simulink model "fillingSystem"  (R2020b)
settings: Solver=VariableStepAuto  StartTime=0.0  StopTime=120  RelTol=1e-3  AbsTol=1e-3
undefined symbols (not defined in the file or in its folder): Sim
libraries: fl_lib x18, nesl_utility x8, pid_lib x1, SimscapeFluids_lib x1, simulink x1
settings Model: PacingRate=4  Creator=luc  LastModifiedBy=luc
settings SolverCC: AutoScaleAbsTol=off
settings DebuggingCC: SymbolicDimsDataTypeCodeGenerationDiagnostic=none
settings SFSimCC: CustomCodeUndefinedFunction=UseInterfaceOnly
settings SimscapeCC: SimscapeLogType=all  SimscapeLogSimulationStatistics=on  SimscapeLogDataHistory=10000

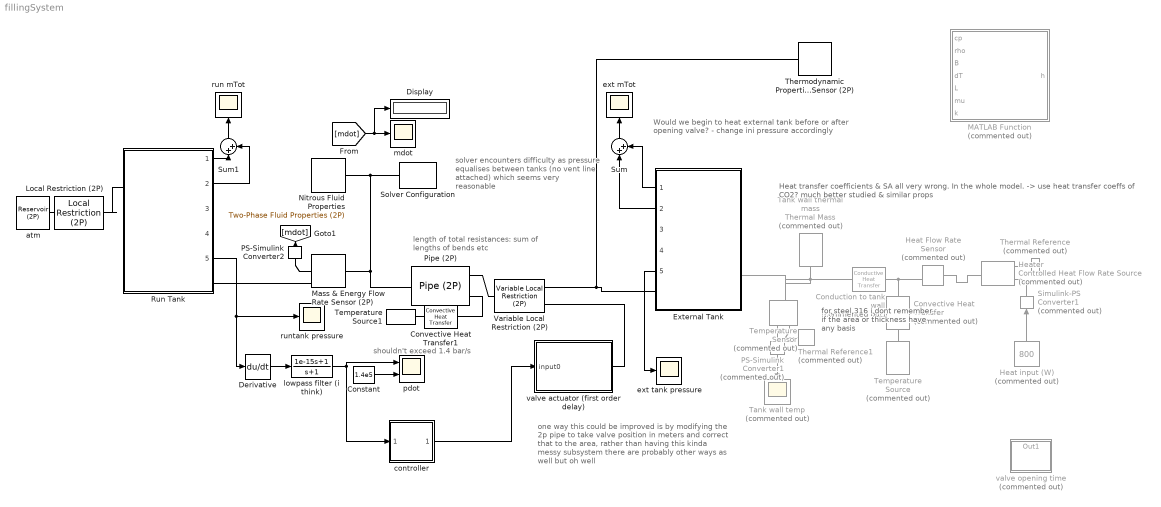
== system fillingSystem ==
  note: one way this could be improved is by modifying
      | the 2p pipe to take valve position in meters and
      | correct that to the area, rather than having this kinda messy subsystem
      |
      | there are probably other ways as well but oh well
  note: for steel 316
      | i dont remember if the area or thickness have any basis
  note: shouldn't exceed 1.4 bar/s
  note: solver encounters difficulty as
      |  pressure equalises between tanks
      | (no vent line attached) which seems
      | very reasonable
  note: Would we begin to heat external tank before or after
      | opening valve? - change ini pressure accordingly
  note: length of total resistances: sum of lengths of bends etc
  note: Heat transfer coefficients & SA all very wrong. In the whole model.
      | -> use heat transfer coeffs of CO2? much better studied & similar props
  Conduction to tank wall : fl_lib/Thermal/Thermal Elements/Conductive Heat Transfer  Commented=on  area=0.63 m^2  thickness=2.2e-3 m  th_cond=16 W/(m*K)  T_specify=off  T_priority=None  T=0 K  T_nominal_specify=off  T_nominal_unit=K  T_nominal_value=1  Q_specify=off  Q_priority=None  Q=0 W  Q_nominal_specify=off  Q_nominal_unit=W  Q_nominal_value=1
  Constant : Constant  Value=1.4e5
  Convective Heat Transfer : fl_lib/Thermal/Thermal Elements/Convective Heat Transfer  Commented=on  area=0.1 m^2  heat_tr_coeff=20 W/(m^2 * K)  T_specify=off  T_priority=None  T=0 K  T_nominal_specify=off  T_nominal_unit=K  T_nominal_value=1  Q_specify=off  Q_priority=None  Q=0 W  Q_nominal_specify=off  Q_nominal_unit=W  Q_nominal_value=1
  Convective Heat Transfer1 : fl_lib/Thermal/Thermal Elements/Convective Heat Transfer  area=3e-4 m^2  heat_tr_coeff=20 W/(m^2 * K)  T_specify=off  T_priority=None  T=0 K  T_nominal_specify=off  T_nominal_unit=K  T_nominal_value=1  Q_specify=off  Q_priority=None  Q=0 W  Q_nominal_specify=off  Q_nominal_unit=W  Q_nominal_value=1
  Derivative : Derivative
  Display : Display
  External Tank : Subsystem  ReferencedSubsystem=Nitrous_Tank_Custom  nitrousLiqConCrossSection=Sim.fillpipe.crossSection  nitrousVapConCrossSection=2e-5  nitrousTankVol=Sim.extTank.volume  initialTankPressure=Sim.extTank.pressure  initialLiqMassFraction=0.7  totalHeatTransferSurfaceArea=6  heatTranferWallToLiq=100  heatTranferWallToVap=15.5
  Heat Flow Rate Sensor : fl_lib/Thermal/Thermal Sensors/Heat Flow Rate Sensor  Commented=on
      settings: SourceProductBaseCode=SS
  Heat input (W) : Constant  Commented=on  Value=800
  Heater : fl_lib/Thermal/Thermal Sources/Controlled Heat Flow Rate Source  Commented=on
  Local Restriction (2P) : fl_lib/Two-Phase Fluid/Elements/Local Restriction (2P)  restriction_area=1e-6 m^2  area=0.01 m^2  Cd=0.64  B_lam=0.999
      settings: SourceProductBaseCode=SS  InternalSimscapePortConfiguration="{\"Bottom\":[],\"Left\":[{\"id\":\"A\",\"label\":\"A\",\"type\":\"foundation.two_phase_fluid.two_phase_fluid\"}],\"Right\":[{\"id\":\"B\",\"label\":\"B\",\"type\":\"foundation.two_phase_fluid.two_phase_fluid\"}],\"Top\":[]}"
  MATLAB Function : MATLAB Function  Commented=on  TreatAsAtomicUnit=on
  Mass & Energy Flow Rate Sensor (2P) : fl_lib/Two-Phase Fluid/Sensors/Mass & Energy Flow Rate Sensor (2P)
      settings: SourceProductBaseCode=SS  InternalSimscapePortConfiguration="{\"Bottom\":[],\"Left\":[{\"id\":\"A\",\"label\":\"A\",\"type\":\"foundation.two_phase_fluid.two_phase_fluid\"}],\"Right\":[{\"id\":\"B\",\"label\":\"B\",\"type\":\"foundation.two_phase_fluid.two_phase_fluid\"},{\"id\":\"M\",\"label\":\"M\",\"type\":\"output\"},{\"id\":\"PHI\",\"label\":\"Phi\",\"type\":\"output\"}],\"Top\":[]}"
  Nitrous Fluid Properties : fl_lib/Two-Phase Fluid/Utilities/Two-Phase Fluid Properties (2P)  u_min=Sim.nitrousFluidTable.u_min kJ/kg  u_max=Sim.nitrousFluidTable.u_max kJ/kg  unorm_liq=Sim.nitrousFluidTable.liquid.unorm  unorm_vap=Sim.nitrousFluidTable.vapor.unorm  p_TLU=Sim.nitrousFluidTable.p MPa  v_liq=Sim.nitrousFluidTable.liquid.v m^3/kg  v_vap=Sim.nitrousFluidTable.vapor.v m^3/kg  s_liq=Sim.nitrousFluidTable.liquid.s kJ/kg/K  s_vap=Sim.nitrousFluidTable.vapor.s kJ/kg/K  T_liq=Sim.nitrousFluidTable.liquid.T K  T_vap=Sim.nitrousFluidTable.vapor.T K  nu_liq=Sim.nitrousFluidTable.liquid.nu mm^2/s  nu_vap=Sim.nitrousFluidTable.vapor.nu mm^2/s  k_liq=Sim.nitrousFluidTable.liquid.k W/(m*K)  k_vap=Sim.nitrousFluidTable.vapor.k W/(m*K)  Pr_liq=Sim.nitrousFluidTable.liquid.Pr  Pr_vap=Sim.nitrousFluidTable.vapor.Pr  u_sat_liq=Sim.nitrousFluidTable.liquid.u_sat kJ/kg  u_sat_vap=Sim.nitrousFluidTable.vapor.u_sat kJ/kg  p_crit=Sim.nitrousFluidTable.p_crit MPa  critical_region=foundation.enum.critical_region.clip  p_crit_fraction=0.12  p_atm=0.101325 MPa  q_rev=0.01 Pa
      settings: SourceProductBaseCode=SS  InternalSimscapePortConfiguration="{\"Bottom\":[],\"Left\":[],\"Right\":[{\"id\":\"A\",\"label\":\"\",\"type\":\"foundation.two_phase_fluid.two_phase_fluid\"}],\"Top\":[]}"
  PS-Simulink Converter1 : nesl_utility/PS-Simulink Converter  Commented=on  PhysicalDomain=network_engine_domain  SubClassName=ps_output  LeftPortType=input  RightPortType=output  PseudoPeriodic=off  Frequencies=[]  Unit=inherit  AffineConversion=off
  PS-Simulink Converter2 : nesl_utility/PS-Simulink Converter  PhysicalDomain=network_engine_domain  SubClassName=ps_output  LeftPortType=input  RightPortType=output  PseudoPeriodic=off  Frequencies=[]  Unit=inherit  AffineConversion=off
  Pipe (2P) : fl_lib/Two-Phase Fluid/Elements/Pipe (2P)  length=1 m  area=Sim.fillpipe.crossSection m^2  Dh=Sim.fillpipe.diameter m  length_add=1 m  roughness=Sim.fillpipe.roughness m  Re_lam=2000  Re_tur=4000  shape_factor=64  Nu_lam=3.66  inertia=simscape.enum.onoff.off  energy_spec=foundation.enum.energy_spec.quality  p_init=1.05e5 Pa  T_init=25 degC  x_init=1  alpha_init=0.1  h_init=1500 kJ/kg  u_init=1500 kJ/kg  mdot_init=0 kg/s  time_constant=0.01 s
      settings: SourceProductBaseCode=SS  InternalSimscapePortConfiguration="{\"Bottom\":[],\"Left\":[{\"id\":\"A\",\"label\":\"A\",\"type\":\"foundation.two_phase_fluid.two_phase_fluid\"},{\"id\":\"H\",\"label\":\"H\",\"type\":\"foundation.thermal.thermal\"}],\"Right\":[{\"id\":\"B\",\"label\":\"B\",\"type\":\"foundation.two_phase_fluid.two_phase_fluid\"}],\"Top\":[]}"
  Run Tank : Subsystem  ReferencedSubsystem=Nitrous_Tank_Custom  nitrousLiqConCrossSection=Sim.fillpipe.crossSection  nitrousVapConCrossSection=2e-5  nitrousTankVol=Sim.runTank.volume  initialTankPressure=Sim.PAmbient  initialLiqMassFraction=0.01  totalHeatTransferSurfaceArea=6  heatTranferWallToLiq=10  heatTranferWallToVap=10
  Simulink-PS Converter1 : nesl_utility/Simulink-PS Converter  Commented=on  PhysicalDomain=network_engine_domain  SubClassName=ps_input  LeftPortType=input  RightPortType=output  PseudoPeriodic=off  Frequencies=[]  NoiseDistribution=none  NoiseParameters=[]  Unit=1  AffineConversion=off  FilteringAndDerivatives=provide  SimscapeFilterOrder=1  InputFilterTimeConstant=0.001  UdotUserProvided=0
  Solver Configuration : nesl_utility/Solver Configuration  PhysicalDomain=network_engine_domain  SubClassName=solver  LeftPortType=input  RightPortType=generic  Tones=[]  Harmonics=[]  SimulateNoise=off  Profile=off  UseLocalSampling=off  EnableSwitchedLinearOptims=on  FrequencyDomain=off  UseCCode=off  RelTol=0.001  AbsTol=1e-06  MinStep=1e-09  ToWorkspace=off  RevertToSquareIcSolve=off  NumHomotopyIterations=100  PhasorMode=off  PhasorModeNumHarmonics=1  DoDC=off  ResidualTolerance=1e-09  UseLocalSolver=off  LocalSolverChoice=NE_BACKWARD_EULER_ADVANCER  LocalSolverSampleTime=0.001  DoFixedCost=off  MaxNonlinIter=3  MaxModeIter=2  ComputeImpulses=off  ImpulseIterations=2  LinearAlgebra=auto  EquationFormulation=NE_TIME_EF  DelaysMemoryBudget=1024  AutomaticFiltering=on  FilteringTimeConstant=0.001  PartitionStorageMethod=AS_NEEDED  PartitionMemoryBudget=1024  PartitionMethod=ROBUST
      settings: SourceProductName=Utilities
  Sum : Sum  Inputs=|++
  Sum1 : Sum  Inputs=|++
  Tank wall thermal mass : fl_lib/Thermal/Thermal Elements/Thermal Mass  Commented=on  mass=6 kg  sp_heat=500 J/kg/K  T_specify=on  T_priority=High  T=300 K  T_nominal_specify=off  T_nominal_unit=K  T_nominal_value=1  Q_specify=off  Q_priority=None  Q=0 W  Q_nominal_specify=off  Q_nominal_unit=W  Q_nominal_value=1
  Tank wall temp : Scope  Commented=on
  Temperature Sensor : fl_lib/Thermal/Thermal Sensors/Temperature Sensor  Commented=on
  Temperature Source : fl_lib/Thermal/Thermal Sources/Temperature Source  Commented=on  temperature=293.15 K
  Temperature Source1 : fl_lib/Thermal/Thermal Sources/Temperature Source  temperature=293.15 K
  Thermal Reference : fl_lib/Thermal/Thermal Elements/Thermal Reference  Commented=on
  Thermal Reference1 : fl_lib/Thermal/Thermal Elements/Thermal Reference  Commented=on
  Thermodynamic Properties Sensor (2P) : fl_lib/Two-Phase Fluid/Sensors/Thermodynamic Properties Sensor (2P)
      settings: SourceProductBaseCode=SS  InternalSimscapePortConfiguration="{\"Bottom\":[],\"Left\":[{\"id\":\"A\",\"label\":\"A\",\"type\":\"foundation.two_phase_fluid.two_phase_fluid\"}],\"Right\":[{\"id\":\"T\",\"label\":\"T\",\"type\":\"output\"},{\"id\":\"H\",\"label\":\"h\",\"type\":\"output\"},{\"id\":\"V\",\"label\":\"v\",\"type\":\"output\"},{\"id\":\"S\",\"label\":\"s\",\"type\":\"output\"}],\"Top\":[]}"
  Variable Local Restriction (2P) : fl_lib/Two-Phase Fluid/Elements/Variable Local Restriction (2P)  min_area=1e-12 m^2  max_area=Sim.controlValve.crossSection m^2  area=Sim.fillpipe.diameter m^2  Cd=0.64  B_lam=0.999
      settings: SourceProductBaseCode=SS  InternalSimscapePortConfiguration="{\"Bottom\":[],\"Left\":[{\"id\":\"A\",\"label\":\"A\",\"type\":\"foundation.two_phase_fluid.two_phase_fluid\"},{\"id\":\"area_in\",\"label\":\"AR\",\"type\":\"input\"}],\"Right\":[{\"id\":\"B\",\"label\":\"B\",\"type\":\"foundation.two_phase_fluid.two_phase_fluid\"}],\"Top\":[]}"
  atm : fl_lib/Two-Phase Fluid/Elements/Reservoir (2P)  pressure_spec=foundation.enum.pressure_spec.atmospheric  reservoir_pressure=0.101325 MPa  energy_spec=foundation.enum.energy_spec.temperature  reservoir_temperature=293.15 K  reservoir_quality=0.5  reservoir_void_fraction=0.5  reservoir_enthalpy=1500 kJ/kg  reservoir_internal_energy=1500 kJ/kg  area_A=5e-7 m^2
      settings: SourceProductBaseCode=SS
  controller : Subsystem
  ext mTot : Scope
  ext tank pressure : Scope
  lowpass filter (i think) : TransferFcn  Numerator=[1e-15, 1]  Denominator=[1 1]
  mdot : Scope
  pdot : Scope  NumInputPorts=2
  run mTot : Scope
  runtank pressure : Scope
  valve actuator (first order delay) : Subsystem
  valve opening time : Subsystem  Commented=on
  wires:
  Heat input (W)/1 -> Simulink-PS Converter1/1
  Sum/1 -> ext mTot/1
  Sum1/1 -> run mTot/1
  PS-Simulink Converter1/1 -> Tank wall temp/1
  PS-Simulink Converter2/1 -> [mdot]
  [mdot] -> Display/1, mdot/1
  Run Tank/5 -> Derivative/1, runtank pressure/1
  External Tank/5 -> ext tank pressure/1
  External Tank/1 -> Sum/2
  External Tank/2 -> Sum/1
  Run Tank/1 -> Sum1/1
  Run Tank/2 -> Sum1/2
  Derivative/1 -> lowpass filter (i think)/1
  lowpass filter (i think)/1 -> controller/1(pdot), pdot/1
  controller/1(Output) -> valve actuator (first order delay)/1(input0)
  Constant/1 -> pdot/2
  connections:
  Variable Local Restriction (2P)/LConn1 -- Thermodynamic Properties Sensor (2P)/LConn1 -- External Tank/RConn1
  Conduction to tank wall/RConn1 -- Temperature Sensor/LConn1 -- External Tank/LConn2 -- Tank wall thermal mass/LConn1
  Convective Heat Transfer/LConn1 -- Heat Flow Rate Sensor/RConn2 -- Conduction to tank wall/LConn1
  Thermal Reference/LConn1 -- Heater/RConn2
  Simulink-PS Converter1/RConn1 -- Heater/RConn1
  Thermal Reference1/LConn1 -- Temperature Sensor/RConn1
  PS-Simulink Converter1/LConn1 -- Temperature Sensor/RConn2
  Convective Heat Transfer/RConn1 -- Temperature Source/LConn1
  Mass & Energy Flow Rate Sensor (2P)/RConn2 -- PS-Simulink Converter2/LConn1
  Convective Heat Transfer1/RConn1 -- Temperature Source1/LConn1
  Pipe (2P)/LConn2 -- Convective Heat Transfer1/LConn1
  Nitrous Fluid Properties/RConn1 -- Solver Configuration/RConn1 -- Pipe (2P)/RConn1 -- Mass & Energy Flow Rate Sensor (2P)/LConn1
  Heat Flow Rate Sensor/LConn1 -- Heater/LConn1
  Pipe (2P)/LConn1 -- Variable Local Restriction (2P)/RConn1
  Run Tank/RConn1 -- Mass & Energy Flow Rate Sensor (2P)/RConn1
  Local Restriction (2P)/LConn1 -- atm/LConn1
  Local Restriction (2P)/RConn1 -- Run Tank/LConn1
  valve actuator (first order delay)/RConn1 -- Variable Local Restriction (2P)/LConn2

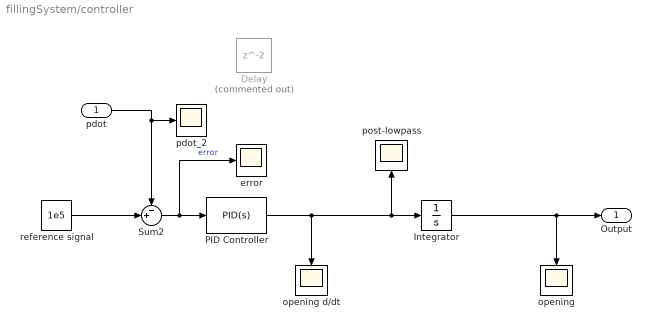
== system fillingSystem/controller ==
  pdot : Inport
  Delay : Delay  Commented=on
  Integrator : Integrator  InitialCondition=0.05  LimitOutput=on  UpperSaturationLimit=1  LowerSaturationLimit=0.05
  PID Controller : pid_lib/PID Controller  Controller=PID  Form=Parallel  TimeDomain=Continuous-time  UseExternalTs=off  SampleTime=-1  IntegratorMethod=Forward Euler  FilterMethod=Forward Euler  ControllerParametersSource=internal  P=2e-5  I=1e-5  D=6e-5  UseFilter=on  N=100  TunerSelectOption=Transfer Function Based (PID Tuner App)  InitialConditionSource=internal  InitialConditionForIntegrator=0  InitialConditionForFilter=0  DifferentiatorICPrevScaledInput=0  ExternalReset=none  TrackingMode=off  Kt=1  LimitOutput=off  SatLimitsSource=internal  UpperSaturationLimit=1  LowerSaturationLimit=0  LinearizeAsGain=on  AntiWindupMode=none  Kb=1  POutMin=[]  POutMax=[]  IOutMin=[]  IOutMax=[]  DOutMin=[]  DOutMax=[]  NOutMin=[]  NOutMax=[]  SumOutMin=[]  SumOutMax=[]  SaturationOutMin=[]  SaturationOutMax=[]  PParamMin=[]  PParamMax=[]  IParamMin=[]  IParamMax=[]  DParamMin=[]  DParamMax=[]  NParamMin=[]  NParamMax=[]  KbParamMin=[]  KbParamMax=[]  KtParamMin=[]  KtParamMax=[]  KbOutMin=[]  KbOutMax=[]  KtOutMin=[]  KtOutMax=[]  IntegratorOutMin=[]  IntegratorOutMax=[]  FilterOutMin=[]  FilterOutMax=[]  SumI1OutMin=[]  SumI1OutMax=[]  SumI2OutMin=[]  SumI2OutMax=[]  SumI3OutMin=[]  SumI3OutMax=[]  SumI4OutMin=[]  SumI4OutMax=[]  SumDOutMin=[]  SumDOutMax=[]  DifferentiatorOutMin=[]  DifferentiatorOutMax=[]  FilterDiffOutCoefMin=[]  FilterDiffOutCoefMax=[]  ReciprocalOutMin=[]  ReciprocalOutMax=[]  SumDenOutMin=[]  SumDenOutMax=[]  SumNumOutMin=[]  SumNumOutMax=[]  DivideOutMin=[]  DivideOutMax=[]  UdiffTsProdOutMin=[]  UdiffTsProdOutMax=[]  NTsProdOutMin=[]  NTsProdOutMax=[]  UintegralTsProdOutMin=[]  UintegralTsProdOutMax=[]  UngainTsProdOutMin=[]  UngainTsProdOutMax=[]  IntegratorContinuousStateAttributes=''  IntegratorStateMustResolveToSignalObject=off  IntegratorRTWStateStorageClass=Auto  FilterContinuousStateAttributes=''  FilterStateMustResolveToSignalObject=off  FilterRTWStateStorageClass=Auto  ParallelPVariant=InternalParameters  IdealPVariant=Disabled  IVariant=InternalParameters  DVariant=InternalParameters  IntegratorVariant=Continuous  SatVariant=Disabled  AWVariant=Passthrough  PCopyVariant=Disabled  TRVariant=Disabled  FdbkBlocksVariant=Forward  IdealPFdbkVariant=Disabled  SatFdbkVariant=Disabled  DerivativeFilterVariant=ContFilter  NVariant=InternalParameters  NCopyVariant=Disabled  FilterICVariant=InternalICsFilter  IntegratorICVariant=InternalICs  ExternalResetVariant=Disabled  TRSumVariant=Passthrough  SumFdbkVariant=Disabled  SumVariant=Sum_PID  TsampFilterVariant=InternalTs  TsampNgainVariant=Passthrough  TsampIntegralVariant=Passthrough  ExternalSaturationOutDataTypeStr=Inherit: Same as second input
  Sum2 : Sum  Inputs=-+|
  error : Scope
  opening : Scope
  opening d/dt : Scope
  pdot_2 : Scope
  post-lowpass : Scope
  reference signal : Constant  Value=1e5
  Output : Outport
  wires:
  reference signal/1 -> Sum2/2
  pdot/1 -> Sum2/1, pdot_2/1
  Sum2/1 -> error/1, PID Controller/1  "error"
  PID Controller/1 -> post-lowpass/1, Integrator/1, opening d/dt/1
  Integrator/1 -> Output/1, opening/1

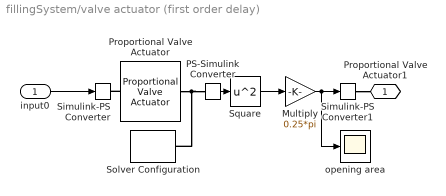
== system fillingSystem/valve actuator (first order delay) ==
  input0 : Inport
  Multiply : Gain  Gain=0.25*pi
  PS-Simulink Converter : nesl_utility/PS-Simulink Converter  PhysicalDomain=network_engine_domain  SubClassName=ps_output  LeftPortType=input  RightPortType=output  PseudoPeriodic=off  Frequencies=[]  Unit=inherit  AffineConversion=off
  Proportional Valve Actuator : SimscapeFluids_lib/Valve Actuators/Proportional Valve Actuator  gain=Sim.controlValve.diameter m  time_constant=8 s  valve_stroke=Sim.controlValve.diameter m
      settings: SourceProductBaseCode=SH  InternalSimscapePortConfiguration="{\"Bottom\":[],\"Left\":[{\"id\":\"A\",\"label\":\"A\",\"type\":\"input\"}],\"Right\":[{\"id\":\"S\",\"label\":\"S\",\"type\":\"output\"}],\"Top\":[]}"
  Simulink-PS Converter : nesl_utility/Simulink-PS Converter  PhysicalDomain=network_engine_domain  SubClassName=ps_input  LeftPortType=input  RightPortType=output  PseudoPeriodic=off  Frequencies=[]  NoiseDistribution=none  NoiseParameters=[]  Unit=1  AffineConversion=off  FilteringAndDerivatives=provide  SimscapeFilterOrder=1  InputFilterTimeConstant=0.001  UdotUserProvided=0
  Simulink-PS Converter1 : nesl_utility/Simulink-PS Converter  PhysicalDomain=network_engine_domain  SubClassName=ps_input  LeftPortType=input  RightPortType=output  PseudoPeriodic=off  Frequencies=[]  NoiseDistribution=none  NoiseParameters=[]  Unit=1  AffineConversion=off  FilteringAndDerivatives=provide  SimscapeFilterOrder=1  InputFilterTimeConstant=0.001  UdotUserProvided=0
  Solver Configuration : nesl_utility/Solver Configuration  PhysicalDomain=network_engine_domain  SubClassName=solver  LeftPortType=input  RightPortType=generic  Tones=[]  Harmonics=[]  SimulateNoise=off  Profile=off  UseLocalSampling=off  EnableSwitchedLinearOptims=on  FrequencyDomain=off  UseCCode=off  RelTol=0.001  AbsTol=1e-06  MinStep=1e-09  ToWorkspace=off  RevertToSquareIcSolve=off  NumHomotopyIterations=100  PhasorMode=off  PhasorModeNumHarmonics=1  DoDC=off  ResidualTolerance=1e-09  UseLocalSolver=off  LocalSolverChoice=NE_BACKWARD_EULER_ADVANCER  LocalSolverSampleTime=0.001  DoFixedCost=off  MaxNonlinIter=3  MaxModeIter=2  ComputeImpulses=off  ImpulseIterations=2  LinearAlgebra=auto  EquationFormulation=NE_TIME_EF  DelaysMemoryBudget=1024  AutomaticFiltering=on  FilteringTimeConstant=0.001  PartitionStorageMethod=AS_NEEDED  PartitionMemoryBudget=1024  PartitionMethod=ROBUST
  Square : Math  Operator=square  SaturateOnIntegerOverflow=on
  opening area : Scope
  Proportional Valve Actuator1 : PMIOPort  Side=Right
  wires:
  input0/1 -> Simulink-PS Converter/1
  Multiply/1 -> opening area/1, Simulink-PS Converter1/1
  Square/1 -> Multiply/1
  PS-Simulink Converter/1 -> Square/1
  connections:
  Proportional Valve Actuator/LConn1 -- Simulink-PS Converter/RConn1
  Proportional Valve Actuator/RConn1 -- Solver Configuration/RConn1 -- PS-Simulink Converter/LConn1
  Simulink-PS Converter1/RConn1 -- Proportional Valve Actuator1/RConn1

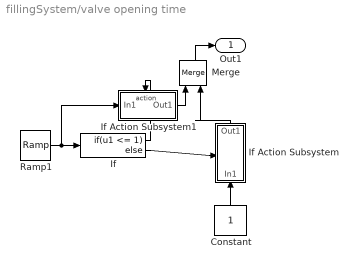
== system fillingSystem/valve opening time ==
  Constant : Constant
  If : If  IfExpression=u1 <= 1
  If Action Subsystem : Subsystem  TreatAsAtomicUnit=on
  If Action Subsystem1 : Subsystem  TreatAsAtomicUnit=on
  Merge : Merge
  Ramp1 : simulink/Sources/Ramp  slope=0.02  start=1  InitialOutput=0.1  VectorParams1D=off
  Out1 : Outport
  wires:
  If Action Subsystem/1(Out1) -> Merge/2
  If/2 -> If Action Subsystem/Action
  Ramp1/1 -> If Action Subsystem1/1(In1), If/1
  Constant/1 -> If Action Subsystem/1(In1)
  Merge/1 -> Out1/1
  If/1 -> If Action Subsystem1/Action
  If Action Subsystem1/1(Out1) -> Merge/1

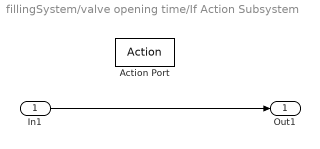
== system fillingSystem/valve opening time/If Action Subsystem ==
  In1 : Inport
  Action Port : ActionPort  ActionPortLabel=else
  Out1 : Outport
  wires:
  In1/1 -> Out1/1

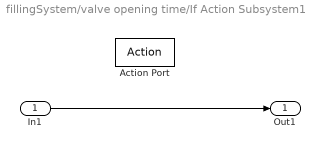
== system fillingSystem/valve opening time/If Action Subsystem1 ==
  In1 : Inport
  Action Port : ActionPort  ActionPortLabel=if(u1 <= 1)
  Out1 : Outport
  wires:
  In1/1 -> Out1/1

== matlab function fillingSystem/MATLAB Function ==
  data: cp input; h output; rho input; B input; dT input; L input; mu input; k input
function h = fcn(cp, rho, B, dT, L, mu, k)
% cp - const pressure heat capacity (kJ / kg K)
% rho - density (kg/m^3)
% B - thermal expansion coeff (1/ K)
% dT - temperature difference (K)
% L - characteristic length (m)
% mu - absolute viscosity (Pa S)
% k - thermal conductivity

% https://web.stanford.edu/~cantwell/Recent_publications/Zimmerman_et_al_AIAA_2013-4045.pdf
% pg 6

    c.air_wall = 0.59;
    c.N2O_wall = 0.021;
    c.liq_vap = 0.15;
    
    n.air_wall = 1/4;
    n.N2O_wall = 2/5;
    n.liq_vap = 1/3;
    
    g = 9.81;
% Rayleigh number
    Ra = (cp .* rho.^2 .* g .* B .* abs(dT) .* L.^3)./(mu .* k);
% Nusselt number correlation, Nu = cRa^n
    Nu = c.N2O_wall .* Ra .* n.N2O_wall;
% h from definition of Nusselt number
    h = Nu .* k./L;
h = h;
